simulink model "axis_integrator"  (Simulink 7.5)
settings: Solver=ode45  StartTime=0.0  StopTime=10.0  RelTol=1e-3
settings Model: Creator=auvt  LastModifiedBy=auvt

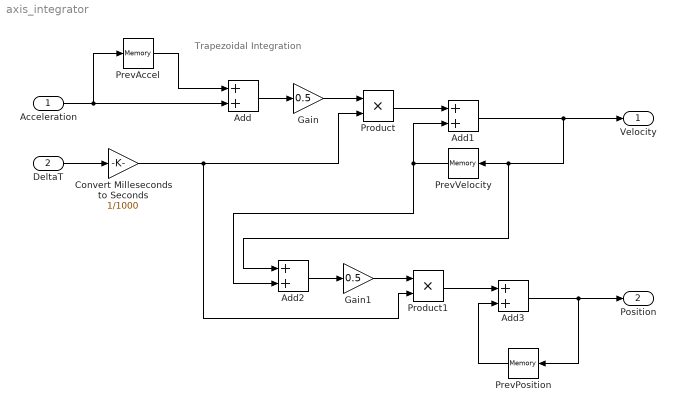
== system axis_integrator ==
  note: Trapezoidal
      | Integration
  Acceleration : Inport  OutDataType=fixdt(1, 16)  OutScaling=2^0
  DeltaT : Inport  Port=2  OutDataType=fixdt(1, 16)  OutScaling=2^0
  Add{,1..3} (4 alike) : Sum  OutDataType=fixdt(1, 16)  OutScaling=2^-10
  Convert Milleseconds to Seconds : Gain  Gain=1/1000  ParameterDataType=fixdt(1, 16)  ParameterScaling=2^0  OutMin=0.001  OutDataType=fixdt(1, 16)  OutScaling=2^0
  Gain : Gain  Gain=0.5  ParameterDataType=fixdt(1, 16)  ParameterScaling=2^0  OutDataType=fixdt(1, 16)  OutScaling=2^0
  Gain1 : Gain  Gain=0.5  ParameterDataType=fixdt(1, 16)  ParameterScaling=2^0  OutDataType=fixdt(1, 16)  OutScaling=2^0
  PrevAccel : Memory
  PrevPosition : Memory
  PrevVelocity : Memory
  Product : Product  OutDataType=fixdt(1, 16)  OutScaling=2^0  RndMeth=Zero
  Product1 : Product  OutDataType=fixdt(1, 16)  OutScaling=2^0  RndMeth=Zero
  Velocity : Outport  OutDataType=fixdt(1, 16)  OutScaling=2^0
  Position : Outport  Port=2  OutDataType=fixdt(1, 16)  OutScaling=2^0
  wires:
  Acceleration/1 -> PrevAccel/1, Add/2
  PrevAccel/1 -> Add/1
  Add/1 -> Gain/1
  Add1/1 -> Velocity/1, PrevVelocity/1, Add2/1
  PrevVelocity/1 -> Add1/2, Add2/2
  Gain/1 -> Product/1
  DeltaT/1 -> Convert Milleseconds to Seconds/1
  Product/1 -> Add1/1
  Convert Milleseconds to Seconds/1 -> Product/2, Product1/2
  Add2/1 -> Gain1/1
  Add3/1 -> PrevPosition/1, Position/1
  PrevPosition/1 -> Add3/2
  Gain1/1 -> Product1/1
  Product1/1 -> Add3/1
